simulink model "Autotrans_shift2"  (R2024a)
settings: Solver=VariableStepAuto  StartTime=0.0  StopTime=35.0  RelTol=0.001
model workspace (MATLAB code in the model file):
  | load sldemo_autotrans_data; %load initial conditions and other necessary data
undefined symbols (not defined in the file or in its folder): converter_data, downtab, emap, Hecate_brake1, Hecate_brake2, Hecate_throttle1, Hecate_throttle2, Hecate_trans, Iei, uptab, vehicledata
(part 2 of 2)

== stateflow chart Autotrans_shift2/RequirementsTable2 ==
  (default) -> (junction 1073744871)
  (junction 1073744871) -> (junction 1073744872) : {
      | % SF_REQ_REV_07
      | }
  (junction 1073744872) -> (junction 1073744874) : {
      | % ExcEvals:
      | % PriEvals:
      | }
  (junction 1073744874) -> (junction 1073744876) : {
      | % HEADER_ASSIGNMENTS
      |
      | }
  (junction 1073744876) -> (junction 1073744878) : {
      | % START_A_4
      | }
  (junction 1073744878) -> (junction 1073744880) : {
      | }
  (junction 1073744880) -> (junction 1073744882)
  (junction 1073744882) -> (junction 1073744884) : {
      | }
  (junction 1073744884) -> (junction 1073744886) : {
      | % END_A_4
      | }
  (junction 1073744886) -> (junction 1073744888) : {
      | % START_R_7
      | }
  (junction 1073744888) -> (junction 1073744890) : {
      | }
  (junction 1073744890) -> (junction 1073744892)
  (junction 1073744892) -> (junction 1073744894) [order 1] : [(((t) >= (0) && (t) <= (20)))]
  (junction 1073744892) -> (junction 1073744900) [order 2]
  (junction 1073744894) -> (junction 1073744896) : {
      | reqtable_postcondition(((speed2)/115 < 1), 'R:1');
      |
      |
      |
      |
      | }
  (junction 1073744896) -> (junction 1073744898) : {
      | }
  (junction 1073744898) -> (junction 1073744900)
  (junction 1073744900) -> (junction 1073744902)
  (junction 1073744902) -> (junction 1073744904) : {
      | % END_R_7
      | }
  (junction 1073744904) -> (junction 1073744906) : {
      | % START_R_19
      | }
  (junction 1073744906) -> (junction 1073744908) : {
      | }
  (junction 1073744908) -> (junction 1073744910)
  (junction 1073744910) -> (junction 1073744912) [order 1] : [(((t) >= (0) && (t) <= (10)))]
  (junction 1073744910) -> (junction 1073744918) [order 2]
  (junction 1073744912) -> (junction 1073744914) : {
      | reqtable_postcondition(((RPM2)/4800 < 1), 'R:2');
      |
      |
      |
      |
      | }
  (junction 1073744914) -> (junction 1073744916) : {
      | }
  (junction 1073744916) -> (junction 1073744918)
  (junction 1073744918) -> (junction 1073744920)
  (junction 1073744920) -> (junction 1073744922) : {
      | % END_R_19
      | }
  (junction 1073744922) -> (junction 1073744924) : {
      | % START_R_34
      | }
  (junction 1073744924) -> (junction 1073744926) : {
      | }
  (junction 1073744926) -> (junction 1073744928)
  (junction 1073744928) -> (junction 1073744930) [order 1] : [((t) == 0)]
  (junction 1073744928) -> (junction 1073744936) [order 2]
  (junction 1073744930) -> (junction 1073744932) : {
      | flaga_out = true;
      | flagb_out = true;
      | flagc_out = true;
      |
      | }
  (junction 1073744932) -> (junction 1073744934) : {
      | }
  (junction 1073744934) -> (junction 1073744936)
  (junction 1073744936) -> (junction 1073744938)
  (junction 1073744938) -> (junction 1073744940) : {
      | % END_R_34
      | }
  (junction 1073744940) -> (junction 1073744942) : {
      | % START_R_22
      | }
  (junction 1073744942) -> (junction 1073744944) : {
      | }
  (junction 1073744944) -> (junction 1073744946)
  (junction 1073744946) -> (junction 1073744948) [order 1] : [(((t) <= (4))) && (speed1 >= 35)]
  (junction 1073744946) -> (junction 1073744954) [order 2]
  (junction 1073744948) -> (junction 1073744950) : {
      | flaga_out = false
      |
      |
      |
      | }
  (junction 1073744950) -> (junction 1073744952) : {
      | }
  (junction 1073744952) -> (junction 1073744954)
  (junction 1073744954) -> (junction 1073744956)
  (junction 1073744956) -> (junction 1073744958) : {
      | % END_R_22
      | }
  (junction 1073744958) -> (junction 1073744960) : {
      | % START_R_67
      | }
  (junction 1073744960) -> (junction 1073744962) : {
      | }
  (junction 1073744962) -> (junction 1073744964)
  (junction 1073744964) -> (junction 1073744966) [order 1] : [((t) > 4 || ((t) > 0 && speed1 < 35))]
  (junction 1073744964) -> (junction 1073744972) [order 2]
  (junction 1073744966) -> (junction 1073744968) : {
      | flaga_out = prev(flaga_out);
      |
      |
      |
      | }
  (junction 1073744968) -> (junction 1073744970) : {
      | }
  (junction 1073744970) -> (junction 1073744972)
  (junction 1073744972) -> (junction 1073744974)
  (junction 1073744974) -> (junction 1073744976) : {
      | % END_R_67
      | }
  (junction 1073744976) -> (junction 1073744978) : {
      | % START_R_52
      | }
  (junction 1073744978) -> (junction 1073744980) : {
      | }
  (junction 1073744980) -> (junction 1073744982)
  (junction 1073744982) -> (junction 1073744984) [order 1] : [duration((((t) <= (30))) && (RPM1 < 3000)) >= 30]
  (junction 1073744982) -> (junction 1073744990) [order 2]
  (junction 1073744984) -> (junction 1073744986) : {
      | reqtable_postcondition((((flaga_in) == (true))), 'R:6');
      |
      |
      |
      |
      | }
  (junction 1073744986) -> (junction 1073744988) : {
      | }
  (junction 1073744988) -> (junction 1073744990)
  (junction 1073744990) -> (junction 1073744992)
  (junction 1073744992) -> (junction 1073744994) : {
      | % END_R_52
      | }
  (junction 1073744994) -> (junction 1073744996) : {
      | % START_R_16
      | }
  (junction 1073744996) -> (junction 1073744998) : {
      | }
  (junction 1073744998) -> (junction 1073745000)
  (junction 1073745000) -> (junction 1073745002) [order 1] : [(((t) <= (8))) && (speed1 >= 52)]
  (junction 1073745000) -> (junction 1073745008) [order 2]
  (junction 1073745002) -> (junction 1073745004) : {
      |
      | flagb_out = false;
      |
      |
      | }
  (junction 1073745004) -> (junction 1073745006) : {
      | }
  (junction 1073745006) -> (junction 1073745008)
  (junction 1073745008) -> (junction 1073745010)
  (junction 1073745010) -> (junction 1073745012) : {
      | % END_R_16
      | }
  (junction 1073745012) -> (junction 1073745014) : {
      | % START_R_70
      | }
  (junction 1073745014) -> (junction 1073745016) : {
      | }
  (junction 1073745016) -> (junction 1073745018)
  (junction 1073745018) -> (junction 1073745020) [order 1] : [((t) > 8 || ((t) > 0 && speed1 < 52))]
  (junction 1073745018) -> (junction 1073745026) [order 2]
  (junction 1073745020) -> (junction 1073745022) : {
      |
      | flagb_out = prev(flagb_out);
      |
      |
      | }
  (junction 1073745022) -> (junction 1073745024) : {
      | }
  (junction 1073745024) -> (junction 1073745026)
  (junction 1073745026) -> (junction 1073745028)
  (junction 1073745028) -> (junction 1073745030) : {
      | % END_R_70
      | }
  (junction 1073745030) -> (junction 1073745032) : {
      | % START_R_55
      | }
  (junction 1073745032) -> (junction 1073745034) : {
      | }
  (junction 1073745034) -> (junction 1073745036)
  (junction 1073745036) -> (junction 1073745038) [order 1] : [duration((((t) <= (30))) && (RPM1 < 2900)) >= 30]
  (junction 1073745036) -> (junction 1073745044) [order 2]
  (junction 1073745038) -> (junction 1073745040) : {
      | reqtable_postcondition((((flagb_in) == (true))), 'R:9');
      |
      |
      |
      |
      | }
  (junction 1073745040) -> (junction 1073745042) : {
      | }
  (junction 1073745042) -> (junction 1073745044)
  (junction 1073745044) -> (junction 1073745046)
  (junction 1073745046) -> (junction 1073745048) : {
      | % END_R_55
      | }
  (junction 1073745048) -> (junction 1073745050) : {
      | % START_R_28
      | }
  (junction 1073745050) -> (junction 1073745052) : {
      | }
  (junction 1073745052) -> (junction 1073745054)
  (junction 1073745054) -> (junction 1073745056) [order 1] : [(((t) <= (20))) && (speed1 >= 65)]
  (junction 1073745054) -> (junction 1073745062) [order 2]
  (junction 1073745056) -> (junction 1073745058) : {
      |
      |
      | flagc_out = false;
      |
      | }
  (junction 1073745058) -> (junction 1073745060) : {
      | }
  (junction 1073745060) -> (junction 1073745062)
  (junction 1073745062) -> (junction 1073745064)
  (junction 1073745064) -> (junction 1073745066) : {
      | % END_R_28
      | }
  (junction 1073745066) -> (junction 1073745068) : {
      | % START_R_73
      | }
  (junction 1073745068) -> (junction 1073745070) : {
      | }
  (junction 1073745070) -> (junction 1073745072)
  (junction 1073745072) -> (junction 1073745074) [order 1] : [((t) > 20 || ((t) > 0 && speed1 < 65))]
  (junction 1073745072) -> (junction 1073745080) [order 2]
  (junction 1073745074) -> (junction 1073745076) : {
      |
      |
      | flagc_out = prev(flagc_out);
      |
      | }
  (junction 1073745076) -> (junction 1073745078) : {
      | }
  (junction 1073745078) -> (junction 1073745080)
  (junction 1073745080) -> (junction 1073745082)
  (junction 1073745082) -> (junction 1073745084) : {
      | % END_R_73
      | }
  (junction 1073745084) -> (junction 1073745086) : {
      | % START_R_58
      | }
  (junction 1073745086) -> (junction 1073745088) : {
      | }
  (junction 1073745088) -> (junction 1073745090)
  (junction 1073745090) -> (junction 1073745092) [order 1] : [duration((((t) <= (30))) && (RPM1 < 3000)) >= 30]
  (junction 1073745090) -> (junction 1073745098) [order 2]
  (junction 1073745092) -> (junction 1073745094) : {
      | reqtable_postcondition((((flagc_in) == (true))), 'R:12');
      |
      |
      |
      |
      | }
  (junction 1073745094) -> (junction 1073745096) : {
      | }
  (junction 1073745096) -> (junction 1073745098)
  (junction 1073745098) -> (junction 1073745100)
  (junction 1073745100) -> (junction 1073745102) : {
      | % END_R_58
      | }
  (junction 1073745102) -> (junction 1073745104) : {
      | % START_R_61
      | }
  (junction 1073745104) -> (junction 1073745106) : {
      | }
  (junction 1073745106) -> (junction 1073745108)
  (junction 1073745108) -> (junction 1073745110) [order 1] : [(((t) >= (0) && (t) <= (50)))]
  (junction 1073745108) -> (junction 1073745116) [order 2]
  (junction 1073745110) -> (junction 1073745112) : {
      | reqtable_postcondition((((speed2) >= (0))) && (((RPM2) >= (0))) && ((flaga_in) == true || (flaga_in) == false) && ((flagb_in) == true || (flagb_in) == false) && ((flagc_in) == true || (flagc_in) == false), 'R:13');
      |
      |
      |
      |
      | }
  (junction 1073745112) -> (junction 1073745114) : {
      | }
  (junction 1073745114) -> (junction 1073745116)
  (junction 1073745116) -> (junction 1073745118)
  (junction 1073745118) -> (junction 1073745120) : {
      | % END_R_61
      | }
  data: RPM1 input; RPM2 input; speed1 input; speed2 input; flaga_out output boolean =true; flagc_out output boolean =true; flagb_out output boolean =true; flaga_in input boolean; flagc_in input boolean; flagb_in input boolean

== stateflow chart Autotrans_shift2/RequirementsTable3 ==
  (default) -> (junction 1073744871)
  (junction 1073744871) -> (junction 1073744872) : {
      | % SF_REQ_REV_07
      | }
  (junction 1073744872) -> (junction 1073744874) : {
      | % ExcEvals:
      | % PriEvals:
      | }
  (junction 1073744874) -> (junction 1073744876) : {
      | % HEADER_ASSIGNMENTS
      |
      | }
  (junction 1073744876) -> (junction 1073744878) : {
      | % START_A_4
      | }
  (junction 1073744878) -> (junction 1073744880) : {
      | }
  (junction 1073744880) -> (junction 1073744882)
  (junction 1073744882) -> (junction 1073744884) : {
      | }
  (junction 1073744884) -> (junction 1073744886) : {
      | % END_A_4
      | }
  (junction 1073744886) -> (junction 1073744888) : {
      | % START_R_7
      | }
  (junction 1073744888) -> (junction 1073744890) : {
      | }
  (junction 1073744890) -> (junction 1073744892)
  (junction 1073744892) -> (junction 1073744894) [order 1] : [(((t) >= (0) && (t) <= (25)))]
  (junction 1073744892) -> (junction 1073744900) [order 2]
  (junction 1073744894) -> (junction 1073744896) : {
      | reqtable_postcondition(((speed2)/125 < 1), 'R:1');
      |
      |
      |
      |
      | }
  (junction 1073744896) -> (junction 1073744898) : {
      | }
  (junction 1073744898) -> (junction 1073744900)
  (junction 1073744900) -> (junction 1073744902)
  (junction 1073744902) -> (junction 1073744904) : {
      | % END_R_7
      | }
  (junction 1073744904) -> (junction 1073744906) : {
      | % START_R_19
      | }
  (junction 1073744906) -> (junction 1073744908) : {
      | }
  (junction 1073744908) -> (junction 1073744910)
  (junction 1073744910) -> (junction 1073744912) [order 1] : [(((t) >= (0) && (t) <= (10)))]
  (junction 1073744910) -> (junction 1073744918) [order 2]
  (junction 1073744912) -> (junction 1073744914) : {
      | reqtable_postcondition(((RPM2)/4800 < 1), 'R:2');
      |
      |
      |
      |
      | }
  (junction 1073744914) -> (junction 1073744916) : {
      | }
  (junction 1073744916) -> (junction 1073744918)
  (junction 1073744918) -> (junction 1073744920)
  (junction 1073744920) -> (junction 1073744922) : {
      | % END_R_19
      | }
  (junction 1073744922) -> (junction 1073744924) : {
      | % START_R_34
      | }
  (junction 1073744924) -> (junction 1073744926) : {
      | }
  (junction 1073744926) -> (junction 1073744928)
  (junction 1073744928) -> (junction 1073744930) [order 1] : [((t) == 0)]
  (junction 1073744928) -> (junction 1073744936) [order 2]
  (junction 1073744930) -> (junction 1073744932) : {
      | flaga_out = true;
      | flagb_out = true;
      | flagc_out = true;
      |
      | }
  (junction 1073744932) -> (junction 1073744934) : {
      | }
  (junction 1073744934) -> (junction 1073744936)
  (junction 1073744936) -> (junction 1073744938)
  (junction 1073744938) -> (junction 1073744940) : {
      | % END_R_34
      | }
  (junction 1073744940) -> (junction 1073744942) : {
      | % START_R_22
      | }
  (junction 1073744942) -> (junction 1073744944) : {
      | }
  (junction 1073744944) -> (junction 1073744946)
  (junction 1073744946) -> (junction 1073744948) [order 1] : [(((t) <= (4))) && (speed1 >= 35)]
  (junction 1073744946) -> (junction 1073744954) [order 2]
  (junction 1073744948) -> (junction 1073744950) : {
      | flaga_out = false
      |
      |
      |
      | }
  (junction 1073744950) -> (junction 1073744952) : {
      | }
  (junction 1073744952) -> (junction 1073744954)
  (junction 1073744954) -> (junction 1073744956)
  (junction 1073744956) -> (junction 1073744958) : {
      | % END_R_22
      | }
  (junction 1073744958) -> (junction 1073744960) : {
      | % START_R_67
      | }
  (junction 1073744960) -> (junction 1073744962) : {
      | }
  (junction 1073744962) -> (junction 1073744964)
  (junction 1073744964) -> (junction 1073744966) [order 1] : [((t) > 4 || ((t) > 0 && speed1 < 35))]
  (junction 1073744964) -> (junction 1073744972) [order 2]
  (junction 1073744966) -> (junction 1073744968) : {
      | flaga_out = prev(flaga_out);
      |
      |
      |
      | }
  (junction 1073744968) -> (junction 1073744970) : {
      | }
  (junction 1073744970) -> (junction 1073744972)
  (junction 1073744972) -> (junction 1073744974)
  (junction 1073744974) -> (junction 1073744976) : {
      | % END_R_67
      | }
  (junction 1073744976) -> (junction 1073744978) : {
      | % START_R_52
      | }
  (junction 1073744978) -> (junction 1073744980) : {
      | }
  (junction 1073744980) -> (junction 1073744982)
  (junction 1073744982) -> (junction 1073744984) [order 1] : [duration((((t) <= (30))) && (RPM1 < 3000)) >= 30]
  (junction 1073744982) -> (junction 1073744990) [order 2]
  (junction 1073744984) -> (junction 1073744986) : {
      | reqtable_postcondition((((flaga_in) == (true))), 'R:6');
      |
      |
      |
      |
      | }
  (junction 1073744986) -> (junction 1073744988) : {
      | }
  (junction 1073744988) -> (junction 1073744990)
  (junction 1073744990) -> (junction 1073744992)
  (junction 1073744992) -> (junction 1073744994) : {
      | % END_R_52
      | }
  (junction 1073744994) -> (junction 1073744996) : {
      | % START_R_16
      | }
  (junction 1073744996) -> (junction 1073744998) : {
      | }
  (junction 1073744998) -> (junction 1073745000)
  (junction 1073745000) -> (junction 1073745002) [order 1] : [(((t) <= (8))) && (speed1 >= 50)]
  (junction 1073745000) -> (junction 1073745008) [order 2]
  (junction 1073745002) -> (junction 1073745004) : {
      |
      | flagb_out = false;
      |
      |
      | }
  (junction 1073745004) -> (junction 1073745006) : {
      | }
  (junction 1073745006) -> (junction 1073745008)
  (junction 1073745008) -> (junction 1073745010)
  (junction 1073745010) -> (junction 1073745012) : {
      | % END_R_16
      | }
  (junction 1073745012) -> (junction 1073745014) : {
      | % START_R_70
      | }
  (junction 1073745014) -> (junction 1073745016) : {
      | }
  (junction 1073745016) -> (junction 1073745018)
  (junction 1073745018) -> (junction 1073745020) [order 1] : [((t) > 8 || ((t) > 0 && speed1 < 50))]
  (junction 1073745018) -> (junction 1073745026) [order 2]
  (junction 1073745020) -> (junction 1073745022) : {
      |
      | flagb_out = prev(flagb_out);
      |
      |
      | }
  (junction 1073745022) -> (junction 1073745024) : {
      | }
  (junction 1073745024) -> (junction 1073745026)
  (junction 1073745026) -> (junction 1073745028)
  (junction 1073745028) -> (junction 1073745030) : {
      | % END_R_70
      | }
  (junction 1073745030) -> (junction 1073745032) : {
      | % START_R_55
      | }
  (junction 1073745032) -> (junction 1073745034) : {
      | }
  (junction 1073745034) -> (junction 1073745036)
  (junction 1073745036) -> (junction 1073745038) [order 1] : [duration((((t) <= (30))) && (RPM1 < 3000)) >= 30]
  (junction 1073745036) -> (junction 1073745044) [order 2]
  (junction 1073745038) -> (junction 1073745040) : {
      | reqtable_postcondition((((flagb_in) == (true))), 'R:9');
      |
      |
      |
      |
      | }
  (junction 1073745040) -> (junction 1073745042) : {
      | }
  (junction 1073745042) -> (junction 1073745044)
  (junction 1073745044) -> (junction 1073745046)
  (junction 1073745046) -> (junction 1073745048) : {
      | % END_R_55
      | }
  (junction 1073745048) -> (junction 1073745050) : {
      | % START_R_28
      | }
  (junction 1073745050) -> (junction 1073745052) : {
      | }
  (junction 1073745052) -> (junction 1073745054)
  (junction 1073745054) -> (junction 1073745056) [order 1] : [(((t) <= (20))) && (speed1 >= 67)]
  (junction 1073745054) -> (junction 1073745062) [order 2]
  (junction 1073745056) -> (junction 1073745058) : {
      |
      |
      | flagc_out = false;
      |
      | }
  (junction 1073745058) -> (junction 1073745060) : {
      | }
  (junction 1073745060) -> (junction 1073745062)
  (junction 1073745062) -> (junction 1073745064)
  (junction 1073745064) -> (junction 1073745066) : {
      | % END_R_28
      | }
  (junction 1073745066) -> (junction 1073745068) : {
      | % START_R_73
      | }
  (junction 1073745068) -> (junction 1073745070) : {
      | }
  (junction 1073745070) -> (junction 1073745072)
  (junction 1073745072) -> (junction 1073745074) [order 1] : [((t) > 20 || ((t) > 0 && speed1 < 67))]
  (junction 1073745072) -> (junction 1073745080) [order 2]
  (junction 1073745074) -> (junction 1073745076) : {
      |
      |
      | flagc_out = prev(flagc_out);
      |
      | }
  (junction 1073745076) -> (junction 1073745078) : {
      | }
  (junction 1073745078) -> (junction 1073745080)
  (junction 1073745080) -> (junction 1073745082)
  (junction 1073745082) -> (junction 1073745084) : {
      | % END_R_73
      | }
  (junction 1073745084) -> (junction 1073745086) : {
      | % START_R_58
      | }
  (junction 1073745086) -> (junction 1073745088) : {
      | }
  (junction 1073745088) -> (junction 1073745090)
  (junction 1073745090) -> (junction 1073745092) [order 1] : [duration((((t) <= (30))) && (RPM1 < 2900)) >= 30]
  (junction 1073745090) -> (junction 1073745098) [order 2]
  (junction 1073745092) -> (junction 1073745094) : {
      | reqtable_postcondition((((flagc_in) == (true))), 'R:12');
      |
      |
      |
      |
      | }
  (junction 1073745094) -> (junction 1073745096) : {
      | }
  (junction 1073745096) -> (junction 1073745098)
  (junction 1073745098) -> (junction 1073745100)
  (junction 1073745100) -> (junction 1073745102) : {
      | % END_R_58
      | }
  (junction 1073745102) -> (junction 1073745104) : {
      | % START_R_61
      | }
  (junction 1073745104) -> (junction 1073745106) : {
      | }
  (junction 1073745106) -> (junction 1073745108)
  (junction 1073745108) -> (junction 1073745110) [order 1] : [(((t) >= (0) && (t) <= (50)))]
  (junction 1073745108) -> (junction 1073745116) [order 2]
  (junction 1073745110) -> (junction 1073745112) : {
      | reqtable_postcondition((((speed2) >= (0))) && (((RPM2) >= (0))) && ((flaga_in) == true || (flaga_in) == false) && ((flagb_in) == true || (flagb_in) == false) && ((flagc_in) == true || (flagc_in) == false), 'R:13');
      |
      |
      |
      |
      | }
  (junction 1073745112) -> (junction 1073745114) : {
      | }
  (junction 1073745114) -> (junction 1073745116)
  (junction 1073745116) -> (junction 1073745118)
  (junction 1073745118) -> (junction 1073745120) : {
      | % END_R_61
      | }
  data: RPM1 input; RPM2 input; speed1 input; speed2 input; flaga_out output boolean =true; flagc_out output boolean =true; flagb_out output boolean =true; flaga_in input boolean; flagc_in input boolean; flagb_in input boolean

== stateflow chart Autotrans_shift2/RequirementsTable4 ==
  (default) -> (junction 1073744871)
  (junction 1073744871) -> (junction 1073744872) : {
      | % SF_REQ_REV_07
      | }
  (junction 1073744872) -> (junction 1073744874) : {
      | % ExcEvals:
      | % PriEvals:
      | }
  (junction 1073744874) -> (junction 1073744876) : {
      | % HEADER_ASSIGNMENTS
      |
      | }
  (junction 1073744876) -> (junction 1073744878) : {
      | % START_A_4
      | }
  (junction 1073744878) -> (junction 1073744880) : {
      | }
  (junction 1073744880) -> (junction 1073744882)
  (junction 1073744882) -> (junction 1073744884) : {
      | }
  (junction 1073744884) -> (junction 1073744886) : {
      | % END_A_4
      | }
  (junction 1073744886) -> (junction 1073744888) : {
      | % START_R_7
      | }
  (junction 1073744888) -> (junction 1073744890) : {
      | }
  (junction 1073744890) -> (junction 1073744892)
  (junction 1073744892) -> (junction 1073744894) [order 1] : [(((t) >= (0) && (t) <= (25)))]
  (junction 1073744892) -> (junction 1073744900) [order 2]
  (junction 1073744894) -> (junction 1073744896) : {
      | reqtable_postcondition(((speed2)/125 < 1), 'R:1');
      |
      |
      |
      |
      | }
  (junction 1073744896) -> (junction 1073744898) : {
      | }
  (junction 1073744898) -> (junction 1073744900)
  (junction 1073744900) -> (junction 1073744902)
  (junction 1073744902) -> (junction 1073744904) : {
      | % END_R_7
      | }
  (junction 1073744904) -> (junction 1073744906) : {
      | % START_R_19
      | }
  (junction 1073744906) -> (junction 1073744908) : {
      | }
  (junction 1073744908) -> (junction 1073744910)
  (junction 1073744910) -> (junction 1073744912) [order 1] : [(((t) >= (0) && (t) <= (8)))]
  (junction 1073744910) -> (junction 1073744918) [order 2]
  (junction 1073744912) -> (junction 1073744914) : {
      | reqtable_postcondition(((RPM2)/4750 < 1), 'R:2');
      |
      |
      |
      |
      | }
  (junction 1073744914) -> (junction 1073744916) : {
      | }
  (junction 1073744916) -> (junction 1073744918)
  (junction 1073744918) -> (junction 1073744920)
  (junction 1073744920) -> (junction 1073744922) : {
      | % END_R_19
      | }
  (junction 1073744922) -> (junction 1073744924) : {
      | % START_R_34
      | }
  (junction 1073744924) -> (junction 1073744926) : {
      | }
  (junction 1073744926) -> (junction 1073744928)
  (junction 1073744928) -> (junction 1073744930) [order 1] : [((t) == 0)]
  (junction 1073744928) -> (junction 1073744936) [order 2]
  (junction 1073744930) -> (junction 1073744932) : {
      | flaga_out = true;
      | flagb_out = true;
      | flagc_out = true;
      |
      | }
  (junction 1073744932) -> (junction 1073744934) : {
      | }
  (junction 1073744934) -> (junction 1073744936)
  (junction 1073744936) -> (junction 1073744938)
  (junction 1073744938) -> (junction 1073744940) : {
      | % END_R_34
      | }
  (junction 1073744940) -> (junction 1073744942) : {
      | % START_R_22
      | }
  (junction 1073744942) -> (junction 1073744944) : {
      | }
  (junction 1073744944) -> (junction 1073744946)
  (junction 1073744946) -> (junction 1073744948) [order 1] : [(((t) <= (4))) && (speed1 >= 32)]
  (junction 1073744946) -> (junction 1073744954) [order 2]
  (junction 1073744948) -> (junction 1073744950) : {
      | flaga_out = false
      |
      |
      |
      | }
  (junction 1073744950) -> (junction 1073744952) : {
      | }
  (junction 1073744952) -> (junction 1073744954)
  (junction 1073744954) -> (junction 1073744956)
  (junction 1073744956) -> (junction 1073744958) : {
      | % END_R_22
      | }
  (junction 1073744958) -> (junction 1073744960) : {
      | % START_R_67
      | }
  (junction 1073744960) -> (junction 1073744962) : {
      | }
  (junction 1073744962) -> (junction 1073744964)
  (junction 1073744964) -> (junction 1073744966) [order 1] : [((t) > 4 || ((t) > 0 && speed1 < 32))]
  (junction 1073744964) -> (junction 1073744972) [order 2]
  (junction 1073744966) -> (junction 1073744968) : {
      | flaga_out = prev(flaga_out);
      |
      |
      |
      | }
  (junction 1073744968) -> (junction 1073744970) : {
      | }
  (junction 1073744970) -> (junction 1073744972)
  (junction 1073744972) -> (junction 1073744974)
  (junction 1073744974) -> (junction 1073744976) : {
      | % END_R_67
      | }
  (junction 1073744976) -> (junction 1073744978) : {
      | % START_R_52
      | }
  (junction 1073744978) -> (junction 1073744980) : {
      | }
  (junction 1073744980) -> (junction 1073744982)
  (junction 1073744982) -> (junction 1073744984) [order 1] : [duration((((t) <= (30))) && (RPM1 < 2900)) >= 30]
  (junction 1073744982) -> (junction 1073744990) [order 2]
  (junction 1073744984) -> (junction 1073744986) : {
      | reqtable_postcondition((((flaga_in) == (true))), 'R:6');
      |
      |
      |
      |
      | }
  (junction 1073744986) -> (junction 1073744988) : {
      | }
  (junction 1073744988) -> (junction 1073744990)
  (junction 1073744990) -> (junction 1073744992)
  (junction 1073744992) -> (junction 1073744994) : {
      | % END_R_52
      | }
  (junction 1073744994) -> (junction 1073744996) : {
      | % START_R_16
      | }
  (junction 1073744996) -> (junction 1073744998) : {
      | }
  (junction 1073744998) -> (junction 1073745000)
  (junction 1073745000) -> (junction 1073745002) [order 1] : [(((t) <= (8))) && (speed1 >= 52)]
  (junction 1073745000) -> (junction 1073745008) [order 2]
  (junction 1073745002) -> (junction 1073745004) : {
      |
      | flagb_out = false;
      |
      |
      | }
  (junction 1073745004) -> (junction 1073745006) : {
      | }
  (junction 1073745006) -> (junction 1073745008)
  (junction 1073745008) -> (junction 1073745010)
  (junction 1073745010) -> (junction 1073745012) : {
      | % END_R_16
      | }
  (junction 1073745012) -> (junction 1073745014) : {
      | % START_R_70
      | }
  (junction 1073745014) -> (junction 1073745016) : {
      | }
  (junction 1073745016) -> (junction 1073745018)
  (junction 1073745018) -> (junction 1073745020) [order 1] : [((t) > 8 || ((t) > 0 && speed1 < 52))]
  (junction 1073745018) -> (junction 1073745026) [order 2]
  (junction 1073745020) -> (junction 1073745022) : {
      |
      | flagb_out = prev(flagb_out);
      |
      |
      | }
  (junction 1073745022) -> (junction 1073745024) : {
      | }
  (junction 1073745024) -> (junction 1073745026)
  (junction 1073745026) -> (junction 1073745028)
  (junction 1073745028) -> (junction 1073745030) : {
      | % END_R_70
      | }
  (junction 1073745030) -> (junction 1073745032) : {
      | % START_R_55
      | }
  (junction 1073745032) -> (junction 1073745034) : {
      | }
  (junction 1073745034) -> (junction 1073745036)
  (junction 1073745036) -> (junction 1073745038) [order 1] : [duration((((t) <= (30))) && (RPM1 < 2900)) >= 30]
  (junction 1073745036) -> (junction 1073745044) [order 2]
  (junction 1073745038) -> (junction 1073745040) : {
      | reqtable_postcondition((((flagb_in) == (true))), 'R:9');
      |
      |
      |
      |
      | }
  (junction 1073745040) -> (junction 1073745042) : {
      | }
  (junction 1073745042) -> (junction 1073745044)
  (junction 1073745044) -> (junction 1073745046)
  (junction 1073745046) -> (junction 1073745048) : {
      | % END_R_55
      | }
  (junction 1073745048) -> (junction 1073745050) : {
      | % START_R_28
      | }
  (junction 1073745050) -> (junction 1073745052) : {
      | }
  (junction 1073745052) -> (junction 1073745054)
  (junction 1073745054) -> (junction 1073745056) [order 1] : [(((t) <= (20))) && (speed1 >= 67)]
  (junction 1073745054) -> (junction 1073745062) [order 2]
  (junction 1073745056) -> (junction 1073745058) : {
      |
      |
      | flagc_out = false;
      |
      | }
  (junction 1073745058) -> (junction 1073745060) : {
      | }
  (junction 1073745060) -> (junction 1073745062)
  (junction 1073745062) -> (junction 1073745064)
  (junction 1073745064) -> (junction 1073745066) : {
      | % END_R_28
      | }
  (junction 1073745066) -> (junction 1073745068) : {
      | % START_R_73
      | }
  (junction 1073745068) -> (junction 1073745070) : {
      | }
  (junction 1073745070) -> (junction 1073745072)
  (junction 1073745072) -> (junction 1073745074) [order 1] : [((t) > 20 || ((t) > 0 && speed1 < 67))]
  (junction 1073745072) -> (junction 1073745080) [order 2]
  (junction 1073745074) -> (junction 1073745076) : {
      |
      |
      | flagc_out = prev(flagc_out);
      |
      | }
  (junction 1073745076) -> (junction 1073745078) : {
      | }
  (junction 1073745078) -> (junction 1073745080)
  (junction 1073745080) -> (junction 1073745082)
  (junction 1073745082) -> (junction 1073745084) : {
      | % END_R_73
      | }
  (junction 1073745084) -> (junction 1073745086) : {
      | % START_R_58
      | }
  (junction 1073745086) -> (junction 1073745088) : {
      | }
  (junction 1073745088) -> (junction 1073745090)
  (junction 1073745090) -> (junction 1073745092) [order 1] : [duration((((t) <= (30))) && (RPM1 < 2900)) >= 30]
  (junction 1073745090) -> (junction 1073745098) [order 2]
  (junction 1073745092) -> (junction 1073745094) : {
      | reqtable_postcondition((((flagc_in) == (true))), 'R:12');
      |
      |
      |
      |
      | }
  (junction 1073745094) -> (junction 1073745096) : {
      | }
  (junction 1073745096) -> (junction 1073745098)
  (junction 1073745098) -> (junction 1073745100)
  (junction 1073745100) -> (junction 1073745102) : {
      | % END_R_58
      | }
  (junction 1073745102) -> (junction 1073745104) : {
      | % START_R_61
      | }
  (junction 1073745104) -> (junction 1073745106) : {
      | }
  (junction 1073745106) -> (junction 1073745108)
  (junction 1073745108) -> (junction 1073745110) [order 1] : [(((t) >= (0) && (t) <= (50)))]
  (junction 1073745108) -> (junction 1073745116) [order 2]
  (junction 1073745110) -> (junction 1073745112) : {
      | reqtable_postcondition((((speed2) >= (0))) && (((RPM2) >= (0))) && ((flaga_in) == true || (flaga_in) == false) && ((flagb_in) == true || (flagb_in) == false) && ((flagc_in) == true || (flagc_in) == false), 'R:13');
      |
      |
      |
      |
      | }
  (junction 1073745112) -> (junction 1073745114) : {
      | }
  (junction 1073745114) -> (junction 1073745116)
  (junction 1073745116) -> (junction 1073745118)
  (junction 1073745118) -> (junction 1073745120) : {
      | % END_R_61
      | }
  data: RPM1 input; RPM2 input; speed1 input; speed2 input; flaga_out output boolean =true; flagc_out output boolean =true; flagb_out output boolean =true; flaga_in input boolean; flagc_in input boolean; flagb_in input boolean

== stateflow chart Autotrans_shift2/RequirementsTable5 ==
  (default) -> (junction 1073744871)
  (junction 1073744871) -> (junction 1073744872) : {
      | % SF_REQ_REV_07
      | }
  (junction 1073744872) -> (junction 1073744874) : {
      | % ExcEvals:
      | % PriEvals:
      | }
  (junction 1073744874) -> (junction 1073744876) : {
      | % HEADER_ASSIGNMENTS
      |
      | }
  (junction 1073744876) -> (junction 1073744878) : {
      | % START_A_4
      | }
  (junction 1073744878) -> (junction 1073744880) : {
      | }
  (junction 1073744880) -> (junction 1073744882)
  (junction 1073744882) -> (junction 1073744884) : {
      | }
  (junction 1073744884) -> (junction 1073744886) : {
      | % END_A_4
      | }
  (junction 1073744886) -> (junction 1073744888) : {
      | % START_R_7
      | }
  (junction 1073744888) -> (junction 1073744890) : {
      | }
  (junction 1073744890) -> (junction 1073744892)
  (junction 1073744892) -> (junction 1073744894) [order 1] : [(((t) >= (0) && (t) <= (25)))]
  (junction 1073744892) -> (junction 1073744900) [order 2]
  (junction 1073744894) -> (junction 1073744896) : {
      | reqtable_postcondition(((speed2)/125 < 1), 'R:1');
      |
      |
      |
      |
      | }
  (junction 1073744896) -> (junction 1073744898) : {
      | }
  (junction 1073744898) -> (junction 1073744900)
  (junction 1073744900) -> (junction 1073744902)
  (junction 1073744902) -> (junction 1073744904) : {
      | % END_R_7
      | }
  (junction 1073744904) -> (junction 1073744906) : {
      | % START_R_19
      | }
  (junction 1073744906) -> (junction 1073744908) : {
      | }
  (junction 1073744908) -> (junction 1073744910)
  (junction 1073744910) -> (junction 1073744912) [order 1] : [(((t) >= (0) && (t) <= (8)))]
  (junction 1073744910) -> (junction 1073744918) [order 2]
  (junction 1073744912) -> (junction 1073744914) : {
      | reqtable_postcondition(((RPM2)/4750 < 1), 'R:2');
      |
      |
      |
      |
      | }
  (junction 1073744914) -> (junction 1073744916) : {
      | }
  (junction 1073744916) -> (junction 1073744918)
  (junction 1073744918) -> (junction 1073744920)
  (junction 1073744920) -> (junction 1073744922) : {
      | % END_R_19
      | }
  (junction 1073744922) -> (junction 1073744924) : {
      | % START_R_34
      | }
  (junction 1073744924) -> (junction 1073744926) : {
      | }
  (junction 1073744926) -> (junction 1073744928)
  (junction 1073744928) -> (junction 1073744930) [order 1] : [((t) == 0)]
  (junction 1073744928) -> (junction 1073744936) [order 2]
  (junction 1073744930) -> (junction 1073744932) : {
      | flaga_out = true;
      | flagb_out = true;
      | flagc_out = true;
      |
      | }
  (junction 1073744932) -> (junction 1073744934) : {
      | }
  (junction 1073744934) -> (junction 1073744936)
  (junction 1073744936) -> (junction 1073744938)
  (junction 1073744938) -> (junction 1073744940) : {
      | % END_R_34
      | }
  (junction 1073744940) -> (junction 1073744942) : {
      | % START_R_22
      | }
  (junction 1073744942) -> (junction 1073744944) : {
      | }
  (junction 1073744944) -> (junction 1073744946)
  (junction 1073744946) -> (junction 1073744948) [order 1] : [(((t) <= (5))) && (speed1 >= 35)]
  (junction 1073744946) -> (junction 1073744954) [order 2]
  (junction 1073744948) -> (junction 1073744950) : {
      | flaga_out = false
      |
      |
      |
      | }
  (junction 1073744950) -> (junction 1073744952) : {
      | }
  (junction 1073744952) -> (junction 1073744954)
  (junction 1073744954) -> (junction 1073744956)
  (junction 1073744956) -> (junction 1073744958) : {
      | % END_R_22
      | }
  (junction 1073744958) -> (junction 1073744960) : {
      | % START_R_67
      | }
  (junction 1073744960) -> (junction 1073744962) : {
      | }
  (junction 1073744962) -> (junction 1073744964)
  (junction 1073744964) -> (junction 1073744966) [order 1] : [((t) > 5 || ((t) > 0 && speed1 < 35))]
  (junction 1073744964) -> (junction 1073744972) [order 2]
  (junction 1073744966) -> (junction 1073744968) : {
      | flaga_out = prev(flaga_out);
      |
      |
      |
      | }
  (junction 1073744968) -> (junction 1073744970) : {
      | }
  (junction 1073744970) -> (junction 1073744972)
  (junction 1073744972) -> (junction 1073744974)
  (junction 1073744974) -> (junction 1073744976) : {
      | % END_R_67
      | }
  (junction 1073744976) -> (junction 1073744978) : {
      | % START_R_52
      | }
  (junction 1073744978) -> (junction 1073744980) : {
      | }
  (junction 1073744980) -> (junction 1073744982)
  (junction 1073744982) -> (junction 1073744984) [order 1] : [duration((((t) <= (30))) && (RPM1 < 3000)) >= 30]
  (junction 1073744982) -> (junction 1073744990) [order 2]
  (junction 1073744984) -> (junction 1073744986) : {
      | reqtable_postcondition((((flaga_in) == (true))), 'R:6');
      |
      |
      |
      |
      | }
  (junction 1073744986) -> (junction 1073744988) : {
      | }
  (junction 1073744988) -> (junction 1073744990)
  (junction 1073744990) -> (junction 1073744992)
  (junction 1073744992) -> (junction 1073744994) : {
      | % END_R_52
      | }
  (junction 1073744994) -> (junction 1073744996) : {
      | % START_R_16
      | }
  (junction 1073744996) -> (junction 1073744998) : {
      | }
  (junction 1073744998) -> (junction 1073745000)
  (junction 1073745000) -> (junction 1073745002) [order 1] : [(((t) <= (10))) && (speed1 >= 50)]
  (junction 1073745000) -> (junction 1073745008) [order 2]
  (junction 1073745002) -> (junction 1073745004) : {
      |
      | flagb_out = false;
      |
      |
      | }
  (junction 1073745004) -> (junction 1073745006) : {
      | }
  (junction 1073745006) -> (junction 1073745008)
  (junction 1073745008) -> (junction 1073745010)
  (junction 1073745010) -> (junction 1073745012) : {
      | % END_R_16
      | }
  (junction 1073745012) -> (junction 1073745014) : {
      | % START_R_70
      | }
  (junction 1073745014) -> (junction 1073745016) : {
      | }
  (junction 1073745016) -> (junction 1073745018)
  (junction 1073745018) -> (junction 1073745020) [order 1] : [((t) > 10 || ((t) > 0 && speed1 < 50))]
  (junction 1073745018) -> (junction 1073745026) [order 2]
  (junction 1073745020) -> (junction 1073745022) : {
      |
      | flagb_out = prev(flagb_out);
      |
      |
      | }
  (junction 1073745022) -> (junction 1073745024) : {
      | }
  (junction 1073745024) -> (junction 1073745026)
  (junction 1073745026) -> (junction 1073745028)
  (junction 1073745028) -> (junction 1073745030) : {
      | % END_R_70
      | }
  (junction 1073745030) -> (junction 1073745032) : {
      | % START_R_55
      | }
  (junction 1073745032) -> (junction 1073745034) : {
      | }
  (junction 1073745034) -> (junction 1073745036)
  (junction 1073745036) -> (junction 1073745038) [order 1] : [duration((((t) <= (30))) && (RPM1 < 3000)) >= 30]
  (junction 1073745036) -> (junction 1073745044) [order 2]
  (junction 1073745038) -> (junction 1073745040) : {
      | reqtable_postcondition((((flagb_in) == (true))), 'R:9');
      |
      |
      |
      |
      | }
  (junction 1073745040) -> (junction 1073745042) : {
      | }
  (junction 1073745042) -> (junction 1073745044)
  (junction 1073745044) -> (junction 1073745046)
  (junction 1073745046) -> (junction 1073745048) : {
      | % END_R_55
      | }
  (junction 1073745048) -> (junction 1073745050) : {
      | % START_R_28
      | }
  (junction 1073745050) -> (junction 1073745052) : {
      | }
  (junction 1073745052) -> (junction 1073745054)
  (junction 1073745054) -> (junction 1073745056) [order 1] : [(((t) <= (22))) && (speed1 >= 65)]
  (junction 1073745054) -> (junction 1073745062) [order 2]
  (junction 1073745056) -> (junction 1073745058) : {
      |
      |
      | flagc_out = false;
      |
      | }
  (junction 1073745058) -> (junction 1073745060) : {
      | }
  (junction 1073745060) -> (junction 1073745062)
  (junction 1073745062) -> (junction 1073745064)
  (junction 1073745064) -> (junction 1073745066) : {
      | % END_R_28
      | }
  (junction 1073745066) -> (junction 1073745068) : {
      | % START_R_73
      | }
  (junction 1073745068) -> (junction 1073745070) : {
      | }
  (junction 1073745070) -> (junction 1073745072)
  (junction 1073745072) -> (junction 1073745074) [order 1] : [((t) > 22 || ((t) > 0 && speed1 < 65))]
  (junction 1073745072) -> (junction 1073745080) [order 2]
  (junction 1073745074) -> (junction 1073745076) : {
      |
      |
      | flagc_out = prev(flagc_out);
      |
      | }
  (junction 1073745076) -> (junction 1073745078) : {
      | }
  (junction 1073745078) -> (junction 1073745080)
  (junction 1073745080) -> (junction 1073745082)
  (junction 1073745082) -> (junction 1073745084) : {
      | % END_R_73
      | }
  (junction 1073745084) -> (junction 1073745086) : {
      | % START_R_58
      | }
  (junction 1073745086) -> (junction 1073745088) : {
      | }
  (junction 1073745088) -> (junction 1073745090)
  (junction 1073745090) -> (junction 1073745092) [order 1] : [duration((((t) <= (30))) && (RPM1 < 3000)) >= 30]
  (junction 1073745090) -> (junction 1073745098) [order 2]
  (junction 1073745092) -> (junction 1073745094) : {
      | reqtable_postcondition((((flagc_in) == (true))), 'R:12');
      |
      |
      |
      |
      | }
  (junction 1073745094) -> (junction 1073745096) : {
      | }
  (junction 1073745096) -> (junction 1073745098)
  (junction 1073745098) -> (junction 1073745100)
  (junction 1073745100) -> (junction 1073745102) : {
      | % END_R_58
      | }
  (junction 1073745102) -> (junction 1073745104) : {
      | % START_R_61
      | }
  (junction 1073745104) -> (junction 1073745106) : {
      | }
  (junction 1073745106) -> (junction 1073745108)
  (junction 1073745108) -> (junction 1073745110) [order 1] : [(((t) >= (0) && (t) <= (50)))]
  (junction 1073745108) -> (junction 1073745116) [order 2]
  (junction 1073745110) -> (junction 1073745112) : {
      | reqtable_postcondition((((speed2) >= (0))) && (((RPM2) >= (0))) && ((flaga_in) == true || (flaga_in) == false) && ((flagb_in) == true || (flagb_in) == false) && ((flagc_in) == true || (flagc_in) == false), 'R:13');
      |
      |
      |
      |
      | }
  (junction 1073745112) -> (junction 1073745114) : {
      | }
  (junction 1073745114) -> (junction 1073745116)
  (junction 1073745116) -> (junction 1073745118)
  (junction 1073745118) -> (junction 1073745120) : {
      | % END_R_61
      | }
  data: RPM1 input; RPM2 input; speed1 input; speed2 input; flaga_out output boolean =true; flagc_out output boolean =true; flagb_out output boolean =true; flaga_in input boolean; flagc_in input boolean; flagb_in input boolean

== stateflow chart Autotrans_shift2/RequirementsTable ==
  (default) -> (junction 1073744871)
  (junction 1073744871) -> (junction 1073744872) : {
      | % SF_REQ_REV_07
      | }
  (junction 1073744872) -> (junction 1073744874) : {
      | % ExcEvals:
      | % PriEvals:
      | }
  (junction 1073744874) -> (junction 1073744876) : {
      | % HEADER_ASSIGNMENTS
      |
      | }
  (junction 1073744876) -> (junction 1073744878) : {
      | % START_A_4
      | }
  (junction 1073744878) -> (junction 1073744880) : {
      | }
  (junction 1073744880) -> (junction 1073744882)
  (junction 1073744882) -> (junction 1073744884) : {
      | }
  (junction 1073744884) -> (junction 1073744886) : {
      | % END_A_4
      | }
  (junction 1073744886) -> (junction 1073744888) : {
      | % START_R_7
      | }
  (junction 1073744888) -> (junction 1073744890) : {
      | }
  (junction 1073744890) -> (junction 1073744892)
  (junction 1073744892) -> (junction 1073744894) [order 1] : [(((t) >= (0) && (t) <= (20)))]
  (junction 1073744892) -> (junction 1073744900) [order 2]
  (junction 1073744894) -> (junction 1073744896) : {
      | reqtable_postcondition(((speed2)/120 < 1), 'R:1');
      |
      |
      |
      |
      | }
  (junction 1073744896) -> (junction 1073744898) : {
      | }
  (junction 1073744898) -> (junction 1073744900)
  (junction 1073744900) -> (junction 1073744902)
  (junction 1073744902) -> (junction 1073744904) : {
      | % END_R_7
      | }
  (junction 1073744904) -> (junction 1073744906) : {
      | % START_R_19
      | }
  (junction 1073744906) -> (junction 1073744908) : {
      | }
  (junction 1073744908) -> (junction 1073744910)
  (junction 1073744910) -> (junction 1073744912) [order 1] : [(((t) >= (0) && (t) <= (10)))]
  (junction 1073744910) -> (junction 1073744918) [order 2]
  (junction 1073744912) -> (junction 1073744914) : {
      | reqtable_postcondition(((RPM2)/4750 < 1), 'R:2');
      |
      |
      |
      |
      | }
  (junction 1073744914) -> (junction 1073744916) : {
      | }
  (junction 1073744916) -> (junction 1073744918)
  (junction 1073744918) -> (junction 1073744920)
  (junction 1073744920) -> (junction 1073744922) : {
      | % END_R_19
      | }
  (junction 1073744922) -> (junction 1073744924) : {
      | % START_R_34
      | }
  (junction 1073744924) -> (junction 1073744926) : {
      | }
  (junction 1073744926) -> (junction 1073744928)
  (junction 1073744928) -> (junction 1073744930) [order 1] : [((t) == 0)]
  (junction 1073744928) -> (junction 1073744936) [order 2]
  (junction 1073744930) -> (junction 1073744932) : {
      | flaga_out = true;
      | flagb_out = true;
      | flagc_out = true;
      |
      | }
  (junction 1073744932) -> (junction 1073744934) : {
      | }
  (junction 1073744934) -> (junction 1073744936)
  (junction 1073744936) -> (junction 1073744938)
  (junction 1073744938) -> (junction 1073744940) : {
      | % END_R_34
      | }
  (junction 1073744940) -> (junction 1073744942) : {
      | % START_R_22
      | }
  (junction 1073744942) -> (junction 1073744944) : {
      | }
  (junction 1073744944) -> (junction 1073744946)
  (junction 1073744946) -> (junction 1073744948) [order 1] : [(((t) <= (4))) && (speed1 >= 35)]
  (junction 1073744946) -> (junction 1073744954) [order 2]
  (junction 1073744948) -> (junction 1073744950) : {
      | flaga_out = false
      |
      |
      |
      | }
  (junction 1073744950) -> (junction 1073744952) : {
      | }
  (junction 1073744952) -> (junction 1073744954)
  (junction 1073744954) -> (junction 1073744956)
  (junction 1073744956) -> (junction 1073744958) : {
      | % END_R_22
      | }
  (junction 1073744958) -> (junction 1073744960) : {
      | % START_R_67
      | }
  (junction 1073744960) -> (junction 1073744962) : {
      | }
  (junction 1073744962) -> (junction 1073744964)
  (junction 1073744964) -> (junction 1073744966) [order 1] : [((t) > 4 || ((t) > 0 && speed1 < 35))]
  (junction 1073744964) -> (junction 1073744972) [order 2]
  (junction 1073744966) -> (junction 1073744968) : {
      | flaga_out = prev(flaga_out);
      |
      |
      |
      | }
  (junction 1073744968) -> (junction 1073744970) : {
      | }
  (junction 1073744970) -> (junction 1073744972)
  (junction 1073744972) -> (junction 1073744974)
  (junction 1073744974) -> (junction 1073744976) : {
      | % END_R_67
      | }
  (junction 1073744976) -> (junction 1073744978) : {
      | % START_R_52
      | }
  (junction 1073744978) -> (junction 1073744980) : {
      | }
  (junction 1073744980) -> (junction 1073744982)
  (junction 1073744982) -> (junction 1073744984) [order 1] : [duration((((t) <= (30))) && (RPM1 < 3000)) >= 30]
  (junction 1073744982) -> (junction 1073744990) [order 2]
  (junction 1073744984) -> (junction 1073744986) : {
      | reqtable_postcondition((((flaga_in) == (true))), 'R:6');
      |
      |
      |
      |
      | }
  (junction 1073744986) -> (junction 1073744988) : {
      | }
  (junction 1073744988) -> (junction 1073744990)
  (junction 1073744990) -> (junction 1073744992)
  (junction 1073744992) -> (junction 1073744994) : {
      | % END_R_52
      | }
  (junction 1073744994) -> (junction 1073744996) : {
      | % START_R_16
      | }
  (junction 1073744996) -> (junction 1073744998) : {
      | }
  (junction 1073744998) -> (junction 1073745000)
  (junction 1073745000) -> (junction 1073745002) [order 1] : [(((t) <= (8))) && (speed1 >= 50)]
  (junction 1073745000) -> (junction 1073745008) [order 2]
  (junction 1073745002) -> (junction 1073745004) : {
      |
      | flagb_out = false;
      |
      |
      | }
  (junction 1073745004) -> (junction 1073745006) : {
      | }
  (junction 1073745006) -> (junction 1073745008)
  (junction 1073745008) -> (junction 1073745010)
  (junction 1073745010) -> (junction 1073745012) : {
      | % END_R_16
      | }
  (junction 1073745012) -> (junction 1073745014) : {
      | % START_R_70
      | }
  (junction 1073745014) -> (junction 1073745016) : {
      | }
  (junction 1073745016) -> (junction 1073745018)
  (junction 1073745018) -> (junction 1073745020) [order 1] : [((t) > 8 || ((t) > 0 && speed1 < 50))]
  (junction 1073745018) -> (junction 1073745026) [order 2]
  (junction 1073745020) -> (junction 1073745022) : {
      |
      | flagb_out = prev(flagb_out);
      |
      |
      | }
  (junction 1073745022) -> (junction 1073745024) : {
      | }
  (junction 1073745024) -> (junction 1073745026)
  (junction 1073745026) -> (junction 1073745028)
  (junction 1073745028) -> (junction 1073745030) : {
      | % END_R_70
      | }
  (junction 1073745030) -> (junction 1073745032) : {
      | % START_R_55
      | }
  (junction 1073745032) -> (junction 1073745034) : {
      | }
  (junction 1073745034) -> (junction 1073745036)
  (junction 1073745036) -> (junction 1073745038) [order 1] : [duration((((t) <= (30))) && (RPM1 < 3000)) >= 30]
  (junction 1073745036) -> (junction 1073745044) [order 2]
  (junction 1073745038) -> (junction 1073745040) : {
      | reqtable_postcondition((((flagb_in) == (true))), 'R:9');
      |
      |
      |
      |
      | }
  (junction 1073745040) -> (junction 1073745042) : {
      | }
  (junction 1073745042) -> (junction 1073745044)
  (junction 1073745044) -> (junction 1073745046)
  (junction 1073745046) -> (junction 1073745048) : {
      | % END_R_55
      | }
  (junction 1073745048) -> (junction 1073745050) : {
      | % START_R_28
      | }
  (junction 1073745050) -> (junction 1073745052) : {
      | }
  (junction 1073745052) -> (junction 1073745054)
  (junction 1073745054) -> (junction 1073745056) [order 1] : [(((t) <= (20))) && (speed1 >= 65)]
  (junction 1073745054) -> (junction 1073745062) [order 2]
  (junction 1073745056) -> (junction 1073745058) : {
      |
      |
      | flagc_out = false;
      |
      | }
  (junction 1073745058) -> (junction 1073745060) : {
      | }
  (junction 1073745060) -> (junction 1073745062)
  (junction 1073745062) -> (junction 1073745064)
  (junction 1073745064) -> (junction 1073745066) : {
      | % END_R_28
      | }
  (junction 1073745066) -> (junction 1073745068) : {
      | % START_R_73
      | }
  (junction 1073745068) -> (junction 1073745070) : {
      | }
  (junction 1073745070) -> (junction 1073745072)
  (junction 1073745072) -> (junction 1073745074) [order 1] : [((t) > 20 || ((t) > 0 && speed1 < 65))]
  (junction 1073745072) -> (junction 1073745080) [order 2]
  (junction 1073745074) -> (junction 1073745076) : {
      |
      |
      | flagc_out = prev(flagc_out);
      |
      | }
  (junction 1073745076) -> (junction 1073745078) : {
      | }
  (junction 1073745078) -> (junction 1073745080)
  (junction 1073745080) -> (junction 1073745082)
  (junction 1073745082) -> (junction 1073745084) : {
      | % END_R_73
      | }
  (junction 1073745084) -> (junction 1073745086) : {
      | % START_R_58
      | }
  (junction 1073745086) -> (junction 1073745088) : {
      | }
  (junction 1073745088) -> (junction 1073745090)
  (junction 1073745090) -> (junction 1073745092) [order 1] : [duration((((t) <= (30))) && (RPM1 < 3000)) >= 30]
  (junction 1073745090) -> (junction 1073745098) [order 2]
  (junction 1073745092) -> (junction 1073745094) : {
      | reqtable_postcondition((((flagc_in) == (true))), 'R:12');
      |
      |
      |
      |
      | }
  (junction 1073745094) -> (junction 1073745096) : {
      | }
  (junction 1073745096) -> (junction 1073745098)
  (junction 1073745098) -> (junction 1073745100)
  (junction 1073745100) -> (junction 1073745102) : {
      | % END_R_58
      | }
  (junction 1073745102) -> (junction 1073745104) : {
      | % START_R_61
      | }
  (junction 1073745104) -> (junction 1073745106) : {
      | }
  (junction 1073745106) -> (junction 1073745108)
  (junction 1073745108) -> (junction 1073745110) [order 1] : [(((t) >= (0) && (t) <= (50)))]
  (junction 1073745108) -> (junction 1073745116) [order 2]
  (junction 1073745110) -> (junction 1073745112) : {
      | reqtable_postcondition((((speed2) >= (0))) && (((RPM2) >= (0))) && ((flaga_in) == true || (flaga_in) == false) && ((flagb_in) == true || (flagb_in) == false) && ((flagc_in) == true || (flagc_in) == false), 'R:13');
      |
      |
      |
      |
      | }
  (junction 1073745112) -> (junction 1073745114) : {
      | }
  (junction 1073745114) -> (junction 1073745116)
  (junction 1073745116) -> (junction 1073745118)
  (junction 1073745118) -> (junction 1073745120) : {
      | % END_R_61
      | }
  data: RPM1 input; RPM2 input; speed1 input; speed2 input; flaga_out output boolean =true; flagc_out output boolean =true; flagb_out output boolean =true; flaga_in input boolean; flagc_in input boolean; flagb_in input boolean
